simulink subsystem "ramp_angle_generator"  (R2019b)
settings: Solver=VariableStepAuto  StartTime=0.0  StopTime=10.0  RelTol=1e-3
settings Model: Creator=andrea  LastModifiedBy=andrea

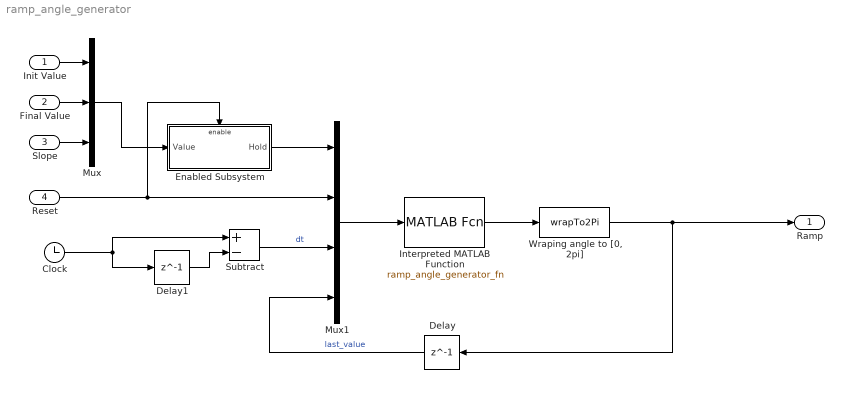
== system ramp_angle_generator ==
  "Init Value " : Inport
  Final Value : Inport  Port=2
  Slope : Inport  Port=3
  Reset : Inport  Port=4
  Clock : Clock
  Delay : Delay  DelayLength=1  SampleTime=0.01
  Delay1 : Delay  DelayLength=1
  Enabled Subsystem : Subsystem  TreatAsAtomicUnit=on
  Interpreted MATLAB Function : MATLABFcn  MATLABFcn=ramp_angle_generator_fn
  Mux : Mux  Inputs=3
  Mux1 : Mux
  Subtract : Sum  Inputs=+-
  "Wraping angle to [0, 2pi]" : MATLABFcn  MATLABFcn=wrapTo2Pi
  Ramp : Outport
  wires:
  "Wraping angle to [0, 2pi]"/1 -> Ramp/1, Delay/1
  Interpreted MATLAB Function/1 -> "Wraping angle to [0, 2pi]"/1
  Subtract/1 -> Mux1/3  "dt"
  Delay1/1 -> Subtract/2
  Clock/1 -> Delay1/1, Subtract/1
  Mux1/1 -> Interpreted MATLAB Function/1
  Enabled Subsystem/1(Hold) -> Mux1/1
  Mux/1 -> Enabled Subsystem/1(Value)
  Final Value/1 -> Mux/2
  Slope/1 -> Mux/3
  Delay/1 -> Mux1/4  "last_value"
  "Init Value "/1 -> Mux/1
  Reset/1 -> Enabled Subsystem/Enable, Mux1/2

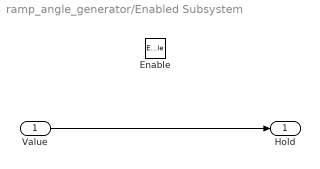
== system ramp_angle_generator/Enabled Subsystem ==
  Value : Inport
  Enable : EnablePort
  Hold : Outport
  wires:
  Value/1 -> Hold/1
